simulink model "cicSimuDetailled"  (R2017a)
settings: Solver=FixedStepAuto  StartTime=0.0  StopTime=14  FixedStep=1  RelTol=1e-3
settings Model: Creator=of-1  LastModifiedBy=of-1
settings DataIOCC: SaveFormat=Array  TimeSaveName=t_out  OutputSaveName=y_out

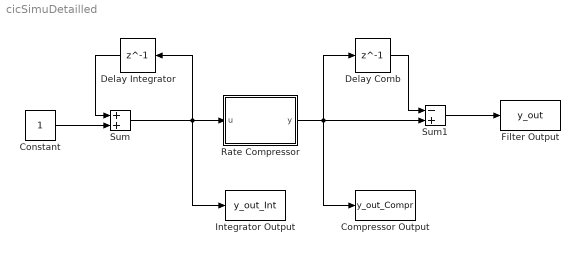
== system cicSimuDetailled ==
  Compressor Output : ToWorkspace  VariableName=y_out_Compr  SampleTime=2
      settings: Save2DSignal=2-D array (concatenate along first dimension)
  Constant : Constant  OutDataTypeStr=fixdt(1,3,0)  SampleTime=1
  Delay Comb : Delay  DelayLength=1  InitialCondition=0  SampleTime=2
  Delay Integrator : Delay  DelayLength=1  InitialCondition=0  SampleTime=1
  Filter Output : ToWorkspace  VariableName=y_out  SampleTime=2
      settings: Save2DSignal=2-D array (concatenate along first dimension)
  Integrator Output : ToWorkspace  VariableName=y_out_Int  SampleTime=1
      settings: Save2DSignal=2-D array (concatenate along first dimension)
  Rate Compressor : MATLAB Function  TreatAsAtomicUnit=on
  Sum : Sum  AccumDataTypeStr=fixdt(1,3,0)  OutDataTypeStr=fixdt(1,3,0)
  Sum1 : Sum  Inputs=-+  AccumDataTypeStr=fixdt(1,3,0)  OutDataTypeStr=fixdt(1,3,0)
  wires:
  Constant/1 -> Sum/2
  Delay Integrator/1 -> Sum/1
  Sum/1 -> Integrator Output/1, Rate Compressor/1(u), Delay Integrator/1
  Delay Comb/1 -> Sum1/1
  Sum1/1 -> Filter Output/1
  Rate Compressor/1(y) -> Compressor Output/1, Delay Comb/1, Sum1/2

== matlab function cicSimuDetailled/Rate Compressor ==
  data: u input; y output
function y = fcn(u)

y = u(1:2:length(u));

end
